simulink model "dsm_3rd_order_ciff_10mhz_model"  (R2024a)
settings: Solver=FixedStepDiscrete  StartTime=0.0  StopTime=0.0002  FixedStep=1e-07  RelTol=1e-3
model workspace (MAT data in the model file):
  A_dsm = [1  0  0; 1  1  -0.00577183233491; 0  1  1]
  B_dsm = [1  -1; 0  0; 0  0]
  C_dsm = [2.3625162736 2.02236426159 0.59546113812]
  D_dsm = [1 0]
  Ts_dsm = 1e-07
  x0_dsm = [0; 0; 0]
settings Model: Creator=sli767  LastModifiedBy=sli767

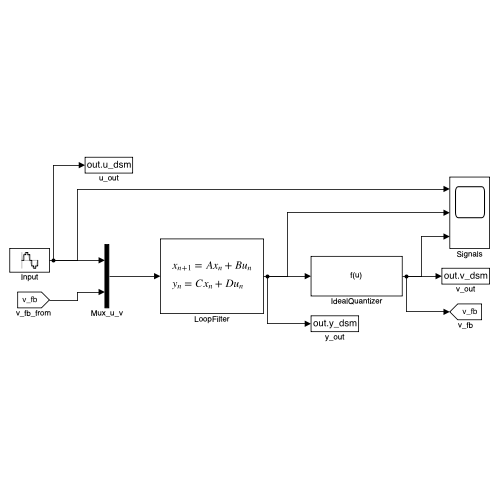
[thumbnail: Simulink's stored preview of the top-level diagram]
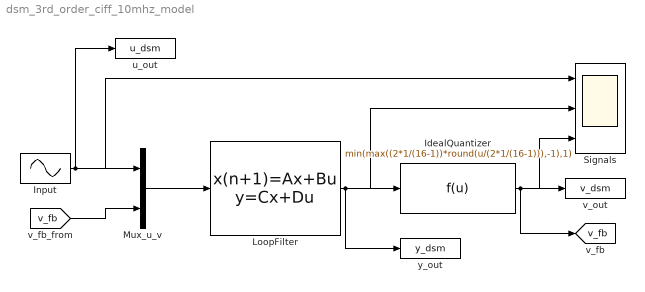
== system dsm_3rd_order_ciff_10mhz_model ==
  IdealQuantizer : Fcn  Expr=min(max((2*1/(16-1))*round(u/(2*1/(16-1))),-1),1)
  Input : Sin  Amplitude=0.5  Frequency=368155.3890925539  SampleTime=1e-07
  LoopFilter : DiscreteStateSpace  A=A_dsm  B=B_dsm  C=C_dsm  D=D_dsm  InitialCondition=x0_dsm  SampleTime=Ts_dsm
  Mux_u_v : Mux  Inputs=2
  Signals : Scope  NumInputPorts=3
  u_out : ToWorkspace  VariableName=u_dsm  SampleTime=-1
  v_out : ToWorkspace  VariableName=v_dsm  SampleTime=-1
  y_out : ToWorkspace  VariableName=y_dsm  SampleTime=-1
  tag scope: v_fb=global
  wires:
  LoopFilter/1 -> y_out/1, IdealQuantizer/1, Signals/2
  Mux_u_v/1 -> LoopFilter/1
  IdealQuantizer/1 -> Signals/3, v_out/1, [v_fb]
  [v_fb] -> Mux_u_v/2
  Input/1 -> u_out/1, Mux_u_v/1, Signals/1
